simulink model "VehicleFollowing"  (R2020b)
settings: Solver=VariableStepAuto  StartTime=0.0  StopTime=50  RelTol=1e-3
undefined symbols (not defined in the file or in its folder): Discrete, Time
libraries: sim3dautolib x3, vrlib x2, simulink x2, ctrlSharedLib x2, mpcadaslib x2, pid_lib x2, sim3dlib x1, robotmobilelib x1
(part 2 of 2)

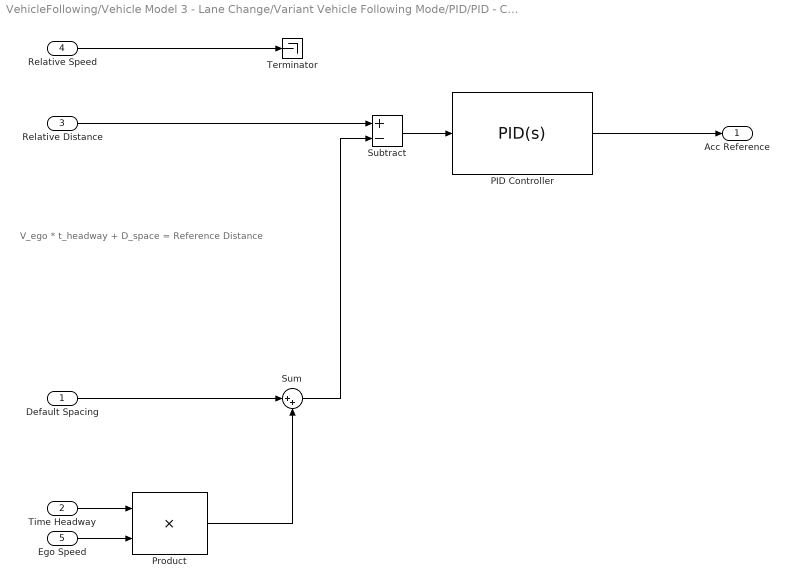
== system VehicleFollowing/Vehicle Model 3 - Lane Change/Variant Vehicle Following Mode/PID/PID - Cruise Control ==
  note: V_ego * t_headway + D_space = Reference Distance
  Default Spacing : Inport
  Time Headway : Inport  Port=2
  Relative Distance : Inport  Port=3
  Relative Speed : Inport  Port=4
  Ego Speed : Inport  Port=5
  PID Controller : pid_lib/PID Controller  Controller=PID  Form=Parallel  TimeDomain=Continuous-time  UseExternalTs=off  SampleTime=-1  IntegratorMethod=Forward Euler  FilterMethod=Forward Euler  ControllerParametersSource=internal  P=2  I=0.04  D=2.1  UseFilter=on  N=230  TunerSelectOption=Transfer Function Based (PID Tuner App)  InitialConditionSource=internal  InitialConditionForIntegrator=0  InitialConditionForFilter=0  DifferentiatorICPrevScaledInput=0  ExternalReset=none  TrackingMode=off  Kt=1  LimitOutput=on  SatLimitsSource=internal  UpperSaturationLimit=2  LowerSaturationLimit=-3  LinearizeAsGain=on  AntiWindupMode=clamping  Kb=1  POutMin=[]  POutMax=[]  IOutMin=[]  IOutMax=[]  DOutMin=[]  DOutMax=[]  NOutMin=[]  NOutMax=[]  SumOutMin=[]  SumOutMax=[]  SaturationOutMin=[]  SaturationOutMax=[]  PParamMin=[]  PParamMax=[]  IParamMin=[]  IParamMax=[]  DParamMin=[]  DParamMax=[]  NParamMin=[]  NParamMax=[]  KbParamMin=[]  KbParamMax=[]  KtParamMin=[]  KtParamMax=[]  KbOutMin=[]  KbOutMax=[]  KtOutMin=[]  KtOutMax=[]  IntegratorOutMin=[]  IntegratorOutMax=[]  FilterOutMin=[]  FilterOutMax=[]  SumI1OutMin=[]  SumI1OutMax=[]  SumI2OutMin=[]  SumI2OutMax=[]  SumI3OutMin=[]  SumI3OutMax=[]  SumI4OutMin=[]  SumI4OutMax=[]  SumDOutMin=[]  SumDOutMax=[]  DifferentiatorOutMin=[]  DifferentiatorOutMax=[]  FilterDiffOutCoefMin=[]  FilterDiffOutCoefMax=[]  ReciprocalOutMin=[]  ReciprocalOutMax=[]  SumDenOutMin=[]  SumDenOutMax=[]  SumNumOutMin=[]  SumNumOutMax=[]  DivideOutMin=[]  DivideOutMax=[]  UdiffTsProdOutMin=[]  UdiffTsProdOutMax=[]  NTsProdOutMin=[]  NTsProdOutMax=[]  UintegralTsProdOutMin=[]  UintegralTsProdOutMax=[]  UngainTsProdOutMin=[]  UngainTsProdOutMax=[]  IntegratorContinuousStateAttributes=''  IntegratorStateMustResolveToSignalObject=off  IntegratorRTWStateStorageClass=Auto  FilterContinuousStateAttributes=''  FilterStateMustResolveToSignalObject=off  FilterRTWStateStorageClass=Auto  ParallelPVariant=InternalParameters  IdealPVariant=Disabled  IVariant=InternalParameters  DVariant=InternalParameters  IntegratorVariant=Continuous  SatVariant=Enabled  AWVariant=ContClampingParallel  PCopyVariant=Disabled  TRVariant=Disabled  FdbkBlocksVariant=Forward  IdealPFdbkVariant=Disabled  SatFdbkVariant=Disabled  DerivativeFilterVariant=ContFilter  NVariant=InternalParameters  NCopyVariant=Disabled  FilterICVariant=InternalICsFilter  IntegratorICVariant=InternalICs  ExternalResetVariant=Disabled  TRSumVariant=Passthrough  SumFdbkVariant=Disabled  SumVariant=Sum_PID  TsampFilterVariant=InternalTs  TsampNgainVariant=Passthrough  TsampIntegralVariant=Passthrough  ExternalSaturationOutDataTypeStr=Inherit: Same as second input
  Product : Product
  Subtract : Sum  Inputs=+-
  Sum : Sum  Inputs=|++
  Terminator : Terminator
  Acc Reference : Outport
  wires:
  Ego Speed/1 -> Product/2
  Time Headway/1 -> Product/1
  Default Spacing/1 -> Sum/1
  Product/1 -> Sum/2
  Sum/1 -> Subtract/2
  Relative Distance/1 -> Subtract/1
  Subtract/1 -> PID Controller/1
  PID Controller/1 -> Acc Reference/1
  Relative Speed/1 -> Terminator/1

== stateflow chart VehicleFollowing/Vehicle Model 3 - Lane Change/Driving Mode Selector ==
  state VehicleFollowing
    entry:
    drivingMode=2;
  state FreeDrive
    entry:
    drivingMode =1;
  state EmergecyBrake
    entry:
    drivingMode=3;
  (default) -> FreeDrive
  VehicleFollowing -> FreeDrive [order 1] : [relativeDistance >50]
  FreeDrive -> VehicleFollowing [order 1] : [relativeDistance <=40]
  FreeDrive -> EmergecyBrake [order 2] : [relativeDistance <=10]
  VehicleFollowing -> EmergecyBrake [order 2] : [relativeDistance <=10]
  EmergecyBrake -> VehicleFollowing : [relativeDistance>15]
  data: relativeDistance input; drivingMode output

== matlab function VehicleFollowing/2D Animation/MATLAB Function ==
  data: V1_Pose input; V2_Pose input; V3_Pose input
function plotVehicle(V1_Pose, V2_Pose, V3_Pose)
%% Clear previous Vehicle
cla;

%% Vehicle 1 - Pose
x1 = V1_Pose(1);
y1 = V1_Pose(2);
yaw1 = V1_Pose(3);

centerP = [x1;y1];

V1_HalfLength = 2; % Length = 4m
V1_HalfWidth = 1; % Width = 2m

% Creating a rectangle
p1 = [V1_HalfLength; V1_HalfWidth];
p2 = [V1_HalfLength; -V1_HalfWidth];
p3 = [-V1_HalfLength; -V1_HalfWidth];
p4 = [-V1_HalfLength; V1_HalfWidth];

% Rotation Matrix
Rmatrix = [cos(yaw1) -sin(yaw1); sin(yaw1) cos(yaw1)];

% Rotated Points
p1r = centerP + Rmatrix*p1;
p2r = centerP + Rmatrix*p2;
p3r = centerP + Rmatrix*p3;
p4r = centerP + Rmatrix*p4;

% Connecting points
Hitbox_V1 = [p1r p2r p3r p4r p1r];

cornersV1_x = transpose(Hitbox_V1(1,:));
cornersV1_y = transpose(Hitbox_V1(2,:));

%% Vehicle 2 - Pose
x2 = V2_Pose(1);
y2 = V2_Pose(2);
yaw2 = V2_Pose(3);

centerP = [x2;y2];

V2_HalfLength = 2; % Length = 4m
V2_HalfWidth = 1; % Width = 2m

% Creating a rectangle
p1 = [V2_HalfLength; V2_HalfWidth];
p2 = [V2_HalfLength; -V2_HalfWidth];
p3 = [-V2_HalfLength; -V2_HalfWidth];
p4 = [-V2_HalfLength; V2_HalfWidth];

% Rotation Matrix

Rmatrix = [cos(yaw2) -sin(yaw2); sin(yaw2) cos(yaw2)];

% Rotated Points
p1r = centerP + Rmatrix*p1;
p2r = centerP + Rmatrix*p2;
p3r = centerP + Rmatrix*p3;
p4r = centerP + Rmatrix*p4;

% Connecting points
Hitbox_V2 = [p1r p2r p3r p4r p1r];

cornersV2_x = transpose(Hitbox_V2(1,:));
cornersV2_y = transpose(Hitbox_V2(2,:));

%% Vehicle 3 - Pose
x3 = V3_Pose(1);
y3 = V3_Pose(2);
yaw3 = V3_Pose(3);

centerP = [x3;y3];

V3_HalfLength = 2; % Length = 4m
V3_HalfWidth = 1; % Width = 2m

% Creating a rectangle
p1 = [V3_HalfLength; V3_HalfWidth];
p2 = [V3_HalfLength; -V3_HalfWidth];
p3 = [-V3_HalfLength; -V3_HalfWidth];
p4 = [-V3_HalfLength; V3_HalfWidth];

% Rotation Matrix
Rmatrix = [cos(yaw3) -sin(yaw3); sin(yaw3) cos(yaw3)];

% Rotated Points
p1r = centerP + Rmatrix*p1;
p2r = centerP + Rmatrix*p2;
p3r = centerP + Rmatrix*p3;
p4r = centerP + Rmatrix*p4;

% Connecting points
Hitbox_V3 = [p1r p2r p3r p4r p1r];

cornersV3_x = transpose(Hitbox_V3(1,:));
cornersV3_y = transpose(Hitbox_V3(2,:));

%% Plot Vehicles and the road
plot(cornersV1_x,cornersV1_y,'g'); %Vehicle 1 rectangle
plot(x1,y1,'*'); %Vehicle 1 center

plot(cornersV2_x,cornersV2_y,'r'); %Vehicle 2 rectangle
plot(x2,y2,'o'); %Vehicle 2 center

plot(cornersV3_x,cornersV3_y,'b'); %Vehicle 3 rectangle
plot(x3,y3,'x'); %Vehicle 3 center

upperLine = plot([0 1000], [5 5], 'Color', 'blue');
midLine = plot([0 1000], [0 0],'--', 'Color', 'blue');
lowerLine = plot([0 1000], [-5 -5], 'Color', 'blue');



% Adjust Axis
axis([x3-40 x3+40 y3-20 y3+20]); % Camera following V3 as ego vehicle

== stateflow chart VehicleFollowing/Vehicle Model 2 - Following/Driving Mode Selector ==
  state VehicleFollowing
    entry:
    drivingMode=2;
  state FreeDrive
    entry:
    drivingMode =1;
  state EmergecyBrake
    entry:
    drivingMode=3;
  (default) -> FreeDrive
  VehicleFollowing -> FreeDrive [order 1] : [relativeDistance >50]
  FreeDrive -> VehicleFollowing [order 1] : [relativeDistance <=40]
  FreeDrive -> EmergecyBrake [order 2] : [relativeDistance <=10]
  VehicleFollowing -> EmergecyBrake [order 2] : [relativeDistance <=10]
  EmergecyBrake -> VehicleFollowing : [relativeDistance>15]
  data: relativeDistance input; drivingMode output
